simulink model "TissueGasExchange"  (R2019b)
settings: Solver=VariableStepAuto  StartTime=0.0  StopTime=10.0  RelTol=1e-3
values from neighbouring files (symbols this model uses):
  CaCO2_IC = 0.487    [xFinalDisease.m]
  CaO2_IC = 0.205    [xFinalDisease.m]
  CvCO2_IC = 0.522    [xFinalDisease.m]
  CvO2_IC = 0.156    [xFinalDisease.m]
  MRCO2 = 0.8*MRO2    (= 3.04)    [xFinalDisease.m]
  MRO2 = 3.80    (= 3.8)    [xFinalDisease.m]
  Tau_LT = 18.0    (= 18)    [xFinalDisease.m]
  Tsamp = 1e-3    (= 0.001)    [xFinalDisease.m]
  VTCO2 = 6000    [xFinalDisease.m]
  VTO2 = 7700    [xFinalDisease.m]
settings Model: Creator=SÜLEYMAN  LastModifiedBy=SÜLEYMAN

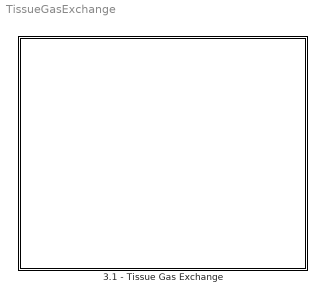
== system TissueGasExchange ==
  3.1 - Tissue Gas Exchange : Subsystem

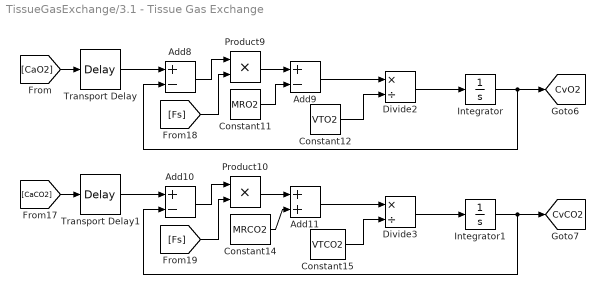
== system TissueGasExchange/3.1 - Tissue Gas Exchange ==
  Add10 : Sum  Inputs=+-
  Add11 : Sum
  Add8 : Sum  Inputs=+-
  Add9 : Sum  Inputs=+-
  Constant11 : Constant  Value=MRO2  SampleTime=Tsamp
  Constant12 : Constant  Value=VTO2  SampleTime=Tsamp
  Constant14 : Constant  Value=MRCO2  SampleTime=Tsamp
  Constant15 : Constant  Value=VTCO2  SampleTime=Tsamp
  Divide2 : Product  Inputs=*/
  Divide3 : Product  Inputs=*/
  Integrator : Integrator  InitialCondition=CvO2_IC
  Integrator1 : Integrator  InitialCondition=CvCO2_IC
  Product10 : Product
  Product9 : Product
  Transport Delay : TransportDelay  DelayTime=Tau_LT  InitialOutput=CaO2_IC
  Transport Delay1 : TransportDelay  DelayTime=Tau_LT  InitialOutput=CaCO2_IC
  tag scope: CvCO2=global, CvO2=global
  wires:
  [Fs] -> Product9/2
  Constant14/1 -> Add11/2
  [CaO2] -> Transport Delay/1
  Divide2/1 -> Integrator/1
  Integrator/1 -> Add8/2, [CvO2]
  Add8/1 -> Product9/1
  Add9/1 -> Divide2/1
  Divide3/1 -> Integrator1/1
  Constant12/1 -> Divide2/2
  Transport Delay/1 -> Add8/1
  Product9/1 -> Add9/1
  Constant11/1 -> Add9/2
  [CaCO2] -> Transport Delay1/1
  Integrator1/1 -> Add10/2, [CvCO2]
  Add11/1 -> Divide3/1
  Product10/1 -> Add11/1
  Transport Delay1/1 -> Add10/1
  Constant15/1 -> Divide3/2
  Add10/1 -> Product10/1
  [Fs] -> Product10/2
